simulink model "ejercicio3"  (R2018a)
settings: Solver=VariableStepAuto  StartTime=0.0  StopTime=20.0  RelTol=1e-3
libraries: simulink x3
settings Model: Creator=OSCAR  LastModifiedBy=OSCAR

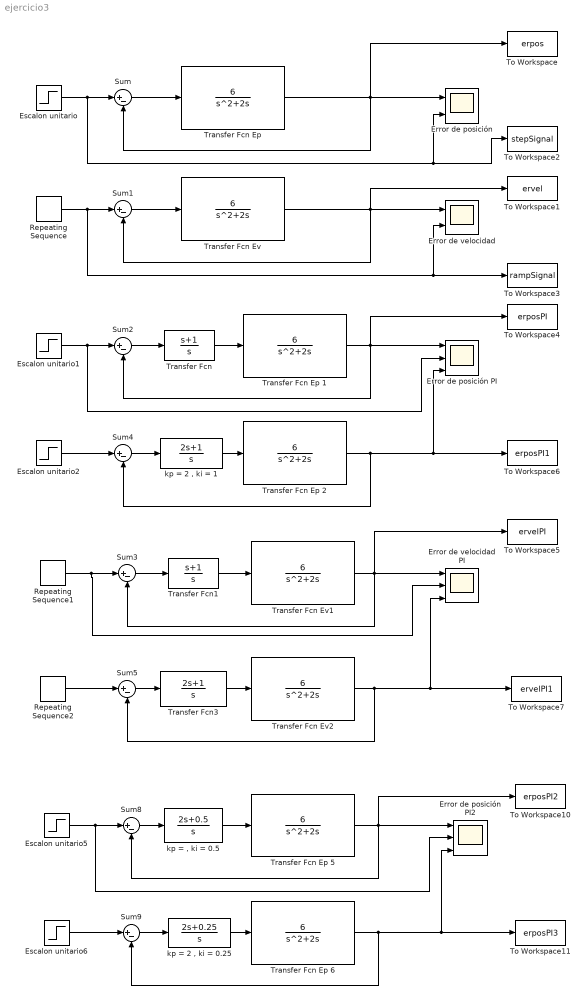
== system ejercicio3 ==
  Error de posición : Scope  NumInputPorts=2
  Error de posición PI : Scope  NumInputPorts=3
  Error de posición PI2 : Scope  NumInputPorts=3
  "Error de velocidad " : Scope  NumInputPorts=2
  Error de velocidad PI : Scope  NumInputPorts=3
  Escalon unitario{,1..2,5..6} (5 alike) : Step  SampleTime=0.01
  Repeating Sequence : simulink/Sources/Repeating Sequence  rep_seq_t=[0 20]  rep_seq_y=[0 20]
  Repeating Sequence1 : simulink/Sources/Repeating Sequence  rep_seq_t=[0 20]  rep_seq_y=[0 20]
  Repeating Sequence2 : simulink/Sources/Repeating Sequence  rep_seq_t=[0 20]  rep_seq_y=[0 20]
  Sum{,1..5,8..9} (8 alike) : Sum  Inputs=|+-
  To Workspace : ToWorkspace  VariableName=erpos  SampleTime=0.01
  To Workspace1 : ToWorkspace  VariableName=ervel  SampleTime=0.01
  To Workspace10 : ToWorkspace  VariableName=erposPI2  SampleTime=0.01
  To Workspace11 : ToWorkspace  VariableName=erposPI3  SampleTime=0.01
  To Workspace2 : ToWorkspace  VariableName=stepSignal  SampleTime=0.01
  To Workspace3 : ToWorkspace  VariableName=rampSignal  SampleTime=0.01
  To Workspace4 : ToWorkspace  VariableName=erposPI  SampleTime=0.01
  To Workspace5 : ToWorkspace  VariableName=ervelPI  SampleTime=0.01
  To Workspace6 : ToWorkspace  VariableName=erposPI1  SampleTime=0.01
  To Workspace7 : ToWorkspace  VariableName=ervelPI1  SampleTime=0.01
  Transfer Fcn : TransferFcn  Numerator=[1 1]  Denominator=[1 0]
  Transfer Fcn Ep {,1..2,5..6} (5 alike) : TransferFcn  Numerator=[6]  Denominator=[1 2 0]
  Transfer Fcn Ev : TransferFcn  Numerator=[6]  Denominator=[1 2 0]
  Transfer Fcn Ev1 : TransferFcn  Numerator=[6]  Denominator=[1 2 0]
  Transfer Fcn Ev2 : TransferFcn  Numerator=[6]  Denominator=[1 2 0]
  Transfer Fcn1 : TransferFcn  Numerator=[1 1]  Denominator=[1 0]
  Transfer Fcn3 : TransferFcn  Numerator=[2 1]  Denominator=[1 0]
  "kp = , ki = 0.5 " : TransferFcn  Numerator=[2 0.5]  Denominator=[1 0]
  "kp = 2 , ki = 0.25" : TransferFcn  Numerator=[2 0.25]  Denominator=[1 0]
  "kp = 2 , ki = 1 " : TransferFcn  Numerator=[2 1]  Denominator=[1 0]
  wires:
  "Transfer Fcn Ep "/1 -> To Workspace/1, Sum/2, Error de posición/1
  Escalon unitario/1 -> To Workspace2/1, Error de posición/2, Sum/1
  Sum/1 -> "Transfer Fcn Ep "/1
  Sum1/1 -> Transfer Fcn Ev/1
  Repeating Sequence/1 -> "Error de velocidad "/2, To Workspace3/1, Sum1/1
  Transfer Fcn Ev/1 -> To Workspace1/1, Sum1/2, "Error de velocidad "/1
  Escalon unitario1/1 -> Error de posición PI/2, Sum2/1
  Transfer Fcn Ep 1/1 -> To Workspace4/1, Sum2/2, Error de posición PI/1
  Sum2/1 -> Transfer Fcn/1
  Transfer Fcn/1 -> Transfer Fcn Ep 1/1
  Repeating Sequence2/1 -> Sum5/1
  Escalon unitario2/1 -> Sum4/1
  Transfer Fcn3/1 -> Transfer Fcn Ev2/1
  "kp = 2 , ki = 1 "/1 -> Transfer Fcn Ep 2/1
  Sum4/1 -> "kp = 2 , ki = 1 "/1
  Sum5/1 -> Transfer Fcn3/1
  Transfer Fcn Ep 2/1 -> Sum4/2, To Workspace6/1, Error de posición PI/3
  Transfer Fcn Ev2/1 -> To Workspace7/1, Error de velocidad PI/3, Sum5/2
  Sum3/1 -> Transfer Fcn1/1
  Transfer Fcn1/1 -> Transfer Fcn Ev1/1
  Transfer Fcn Ev1/1 -> To Workspace5/1, Error de velocidad PI/1, Sum3/2
  Repeating Sequence1/1 -> Error de velocidad PI/2, Sum3/1
  Transfer Fcn Ep 5/1 -> To Workspace10/1, Sum8/2, Error de posición PI2/1
  Sum9/1 -> "kp = 2 , ki = 0.25"/1
  Sum8/1 -> "kp = , ki = 0.5 "/1
  Escalon unitario6/1 -> Sum9/1
  Escalon unitario5/1 -> Error de posición PI2/2, Sum8/1
  "kp = , ki = 0.5 "/1 -> Transfer Fcn Ep 5/1
  Transfer Fcn Ep 6/1 -> Sum9/2, To Workspace11/1, Error de posición PI2/3
  "kp = 2 , ki = 0.25"/1 -> Transfer Fcn Ep 6/1
